simulink model "regler_strecke"  (Simulink 7.0)
settings: Solver=ode4  SolverMode=SingleTasking  StartTime=0.0  StopTime=10  FixedStep=0.001  RelTol=1e-3
undefined symbols (not defined in the file): National_Instruments, PCI
libraries: rtwinlib x2
settings Model: Creator=Admin  LastModifiedBy=Student  SimulationMode=external  ExtModeTrigDuration=1000000
settings OptimizationCC: InlineInvariantSignals=on
settings DebuggingCC: SaveWithParameterizedLinksMsg=none  SignalResolutionControl=TryResolveAllWithWarning  MultiTaskDSMMsg=warning  MultiTaskCondExecSysMsg=none  StrictBusMsg=None
settings RTWCC: SystemTargetFile=rtwin.tlc  TemplateMakefile=rtwin.tmf  Description=Real-Time Windows Target  ProcessScript=rtwin_make_rtw_hook  IncludeERTFirstTime=on
settings RTWinTargetCC: TargetFcnLib=ansi_tfl_tmw.mat  GenFloatMathFcnCalls=ANSI_C  ModelReferenceCompliant=off  CompOptLevelCompliant=off  PortableWordSizes=off  CCOptimize=on

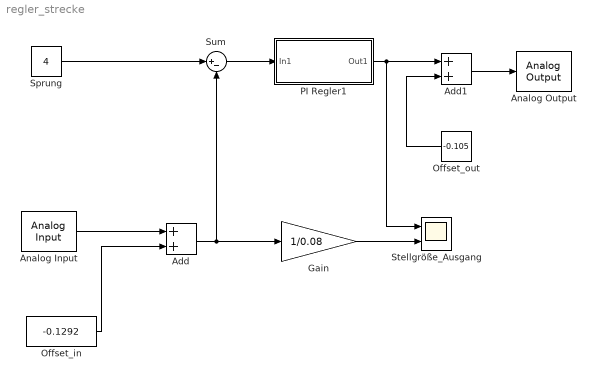
== system regler_strecke ==
  Add : Sum  OutDataType=sfix(16)  OutScaling=2^-10
  Add1 : Sum  OutDataType=sfix(16)  OutScaling=2^-10
  Analog Input : rtwinlib/Analog Input  SampleTime=0.001  DrvName=National_Instruments/PCI-6025E  DrvAddress=4294967295  DrvOptions=[0 1 0 0 0 0]  Channels=1  RangeMode=1  VoltRange=1  DataType=1
      settings: AttributesFormatString=National Instruments\nPCI-6025E [auto]
  Analog Output : rtwinlib/Analog Output  SampleTime=0.001  DrvName=National_Instruments/PCI-6025E  DrvAddress=4294967295  DrvOptions=[0 1 0 0 0 0]  Channels=1  RangeMode=1  VoltRange=1  InitialValue=0  FinalValue=0
      settings: AttributesFormatString=National Instruments\nPCI-6025E [auto]
  Gain : Gain  Gain=1/0.08  ParameterDataType=sfix(16)  ParameterScaling=2^0  OutDataType=sfix(16)  OutScaling=2^0
  Offset_in : Constant  Value=-0.1292  OutDataType=sfix(16)  OutScaling=2^0  SampleTime=-1
  Offset_out : Constant  Orientation=left  Value=-0.105  OutDataType=sfix(16)  OutScaling=2^0  SampleTime=-1
  PI Regler1 : Subsystem
  Sprung : Constant  Value=4  OutDataType=sfix(16)  OutScaling=2^0  SampleTime=-1
  Stellgröße_Ausgang : Scope  NumInputPorts=2
      settings: TimeRange=1  YMin=2.75~27.5  YMax=4.75~55
  Sum : Sum  Inputs=|+-  OutDataType=sfix(16)  OutScaling=2^0
  wires:
  Analog Input/1 -> Add/1
  Offset_in/1 -> Add/2
  Add/1 -> Sum/2, Gain/1
  Sprung/1 -> Sum/1
  Sum/1 -> PI Regler1/1(In1)
  PI Regler1/1(Out1) -> Add1/1, Stellgröße_Ausgang/1
  Offset_out/1 -> Add1/2
  Add1/1 -> Analog Output/1
  Gain/1 -> Stellgröße_Ausgang/2

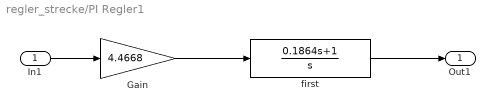
== system regler_strecke/PI Regler1 ==
  In1 : Inport  OutDataType=sfix(16)  OutScaling=2^0
  Gain : Gain  Gain=4.4668  ParameterDataType=sfix(16)  ParameterScaling=2^0  OutDataType=sfix(16)  OutScaling=2^0
  first : TransferFcn  Numerator=[0.1864 1]  Denominator=[1 0]
  Out1 : Outport  OutDataType=sfix(16)  OutScaling=2^0
  wires:
  In1/1 -> Gain/1
  first/1 -> Out1/1
  Gain/1 -> first/1
